simulink model "PVmpptBuckConverter"  (R2020b)
settings: Solver=FixedStepDiscrete  StartTime=0.0  StopTime=0.5  FixedStep=1e-6  RelTol=1e-3
values from neighbouring files (symbols this model uses):
  C = (Iripp)/(8*fs*Vripp)    (= 0.00025)    [BuckConverterCalculos.m]
  L = (Vout* (Vin-Vout))/ (Iripp*fs *Vin)    (= 0.0714285714286)    [BuckConverterCalculos.m]
  Ts = 1e-6    (= 1e-06)    [BuckConverterCalculos.m]
undefined symbols (not defined in the file or in its folder): Ion, Lithium
libraries: powerlib x6, powerlib_meascontrol x2, electricdrivelib x1, re_lib x1
settings Model: Creator=User  LastModifiedBy=User

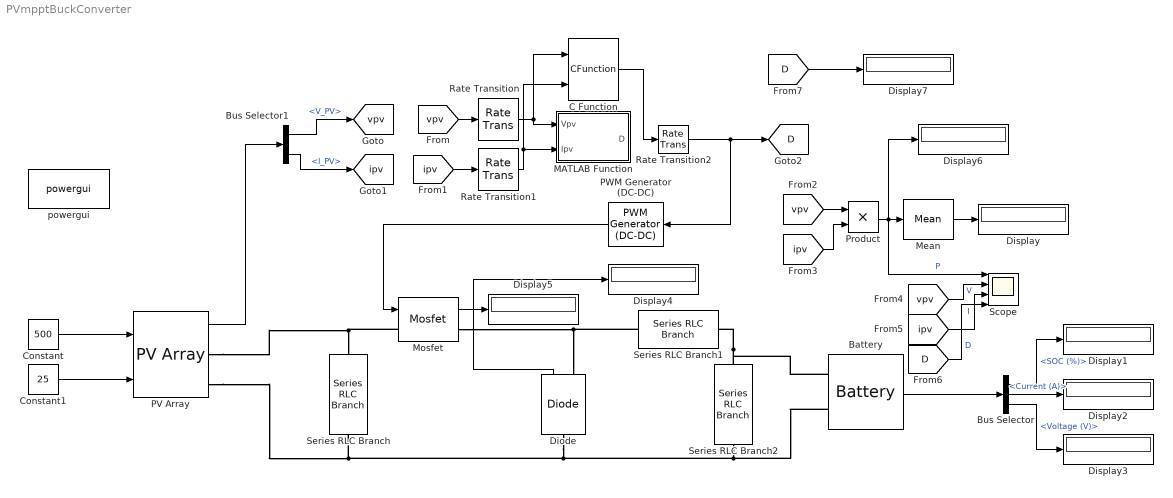
== system PVmpptBuckConverter ==
  Battery : electricdrivelib/Extra Sources/Battery  BatType=Lithium-Ion  ShowTempParam=off  ThermalPreset=no  ShowAgeParam=off  NomV=5  NomQ=50  SOC=45  Batt_Tr=1  PresetModel=on  MaxQ=50  MinV=3.75  FullV=5.8199  Dis_rate=21.7391  R=0.001  Normal_OP=45.2174  expZone="[5.4019      2.4565]"  current=[6.5 13 32.5]  Units=Time  Tci=20  NomT=20  T2=-30  MaxQ2=4.8  FullV2=7.1  Normal_OP2=5.655  expZone2="[6.58           1]"  Rca=0.6  ti=2000  Dp=0  Neq0=0  Tsim=1e6  Ta1=25  Qeol=5.4*0.9  Reol=0.013333*1.2  Char_age=[2.3478, 3]  Dis_age=[2.3478, 10]  N1=1500  N2=10500  N3=1000  N4=1400  Ta2=45  N5=950
  Bus Selector : BusSelector  OutputSignals=SOC (%),Current (A),Voltage (V)
  Bus Selector1 : BusSelector  OutputSignals=V_PV,I_PV
  C Function : CFunction  OutputCode=|  StartCode=|
      OutputCode=|
      | double Ppv = Vpv * Ipv;
      |     double delP = Ppv - Pprev;
      |     double delV = Vpv - Vprev;
      |     
      |     if (delP != 0) {
      |         if (delP > 0) {
      |             if (delV > 0) {
      |                 D = Dprev - deltaD;
      |             } else {
      |                 D = Dprev + deltaD;
      |             }
      |         } else {
      |             if (delV > 0) {
      |                 D = Dprev + deltaD;
      |             } else {
      |                 D = Dprev - deltaD;
      |             }
      |         }
      |     } else {
      |         D = Dprev;
      |     }
      |     if ((D > Dmax) || (D < Dmin)) {
      |         D = Dprev;
      |     }
      |     
      |     Dprev = D;
      |     Pprev = Ppv;
      |     Vprev = Vpv;
      StartCode=|
      | Dmin = 0.05;
      | Dmax = 0.95;
      | Dprev = 0.95;
      | Vprev = 0;
      | Pprev = 0;
      | deltaD = 0.02;
  Constant : Constant  Value=500  SampleTime=Ts
  Constant1 : Constant  Value=25  SampleTime=Ts
  Diode : powerlib/Power Electronics/Diode  Ron=0.001  Lon=0  Vf=0.8  IC=0  UseSnubber=0  Rs=500  Cs=250e-9  Measurements=on
  Display{,1..7} (8 alike) : Display
  MATLAB Function : MATLAB Function  TreatAsAtomicUnit=on
  Mean : powerlib_meascontrol/Measurements/Mean  Freq=60  Vinit=0  Ts=Ts
  Mosfet : powerlib/Power Electronics/Mosfet  Ron=0.1  Lon=0  Rd=0.01  Vfd=0  IC=0  Rs=1e5  Cs=inf  Measurements=on
  PV Array : re_lib/Solar/PV Array  Npar=1  Nser=1  PlotType=array @ 25 deg.C & specified irradiances  S_vec="[ 1000  500  100 ]"  Temp_C_vec="[ 45 25  ]"  ModuleName=User-defined  PlotWhenSelected=off  Pm=5.075  Ncell=36  Voc=22  Isc=0.32  Vm=17.5  Im=0.29  beta_Voc_pc=-0.291  alpha_Isc_pc=0.013301  beta_Voc=-0.06402  alpha_Isc=4.2563e-05  IL=0.32489  I0=6.8687e-13  nI=0.88738  Rsh=903.5702  Rs=6.9286  RobustModel=off  RobustCellTemperature=313.3991  BAL=on  Tc=1e-6  Tfilter=5e-5
  PWM Generator (DC-DC) : powerlib_meascontrol/Pulse & Signal Generators/PWM Generator (DC-DC)  Fsw=500  Ts=Ts
  Product : Product
  Rate Transition : RateTransition  OutPortSampleTime=Ts_control
  Rate Transition1 : RateTransition  OutPortSampleTime=Ts_control
  Rate Transition2 : RateTransition  OutPortSampleTime=Ts
  Scope : Scope  NumInputPorts=4
  Series RLC Branch : powerlib/Elements/Series RLC Branch  LConnTagsString=__new0  RConnTagsString=__new0  BranchType=RC  Resistance=0.001  Inductance=1e-3  SetiL0=off  InitialCurrent=0  Capacitance=C*4  Setx0=off  InitialVoltage=0  Measurements=None
  Series RLC Branch1 : powerlib/Elements/Series RLC Branch  LConnTagsString=__new0  RConnTagsString=__new0  BranchType=L  Resistance=0.001  Inductance=L  SetiL0=off  InitialCurrent=0  Capacitance=2.5e-5  Setx0=off  InitialVoltage=0  Measurements=None
  Series RLC Branch2 : powerlib/Elements/Series RLC Branch  LConnTagsString=__new0  RConnTagsString=__new0  BranchType=C  Resistance=0.001  Inductance=0.0036  SetiL0=off  InitialCurrent=0  Capacitance=C  Setx0=off  InitialVoltage=0  Measurements=None
  powergui : powerlib/powergui  Priority=1  SimulationMode=Discrete  SampleTime=Ts  frequency=60  Iterations=50  frequencyindice=0  Pbase=100e6  ErrMax=1e-4  UnitsV=kV  UnitsW=MW  buscounter=0  FunctionMessages=off  echomessages=off  EnableUseOfTLC=off  CurrentSourceSwitches=off  DisableSnubberDevices=off  DisableRonSwitches=off  DisableVfSwitches=off  DisplayEquations=off  AutomaticDiscreteSolvers=off  SolverType=Tustin/Backward Euler (TBE)  Interpol=off  ExternalGateDelay=off  methode=off  Ts=100  x0status=blocks  SPID=on  SwTol=0  HookPort=off  NonlinearTolerance=1e-4  nMaxIteration=100  ContinueOnMaxIteration=off  RestoreLinks=warning  ResistiveCurrentMeasurement=off  Frange=[0:2:500]  Ylog=off  Xlog=on  ShowGrid=off  save=off  variable=ZData  structure=0  ZoomFFT=off  StartTime=0.0  cycles=1  DisplayStyle=1  fundamental=60  FreqAxis=off  MaxFrequency=1000  frequencyindicesteady=1  RmsSteady=1  display=off
  tag scope: D=global, ipv=global, vpv=global
  wires:
  Constant/1 -> PV Array/1
  Constant1/1 -> PV Array/2
  Battery/1 -> Bus Selector/1
  PV Array/1 -> Bus Selector1/1
  Bus Selector1/1 -> [vpv]  "<V_PV>"
  Bus Selector1/2 -> [ipv]  "<I_PV>"
  [vpv] -> Rate Transition/1
  [ipv] -> Rate Transition1/1
  [vpv] -> Product/1
  [ipv] -> Product/2
  Bus Selector/1 -> Display1/1  "<SOC (%)>"
  Bus Selector/2 -> Display2/1  "<Current (A)>"
  Bus Selector/3 -> Display3/1  "<Voltage (V)>"
  Diode/1 -> Display4/1
  Mosfet/1 -> Display5/1
  Product/1 -> Display6/1, Scope/1, Mean/1  "P"
  Mean/1 -> Display/1
  [vpv] -> Scope/2  "V"
  [ipv] -> Scope/3  "I"
  PWM Generator (DC-DC)/1 -> Mosfet/1
  Rate Transition2/1 -> [D], PWM Generator (DC-DC)/1
  Rate Transition/1 -> C Function/1, MATLAB Function/1(Vpv)
  Rate Transition1/1 -> MATLAB Function/2(Ipv), C Function/2
  [D] -> Scope/4  "D"
  [D] -> Display7/1
  C Function/1 -> Rate Transition2/1
  connections:
  PV Array/RConn1 -- Mosfet/LConn1 -- Series RLC Branch/LConn1
  PV Array/RConn2 -- Battery/LConn2 -- Series RLC Branch2/RConn1 -- Diode/LConn1 -- Series RLC Branch/RConn1
  Mosfet/RConn1 -- Series RLC Branch1/LConn1 -- Diode/RConn1
  Series RLC Branch2/LConn1 -- Battery/LConn1 -- Series RLC Branch1/RConn1

== matlab function PVmpptBuckConverter/MATLAB Function ==
  data: Vpv input; D output; Ipv input
function D = mpptm(Vpv,Ipv)

Dmin = 0.05;
Dmax = 0.95;
persistent Dprev Pprev Vprev ;

if isempty(Dprev)
    Dprev = 0.95;
    Vprev = 0;
    Pprev = 0;
end
%initialize parameters
deltaD = 0.02;

% initalize measured array power
Ppv = Vpv*Ipv;

if((Ppv - Pprev) ~= 0) 
    if((Ppv - Pprev) > 0) 
        if((Vpv-Vprev) > 0) 
            D = Dprev - deltaD;
        else
            D = Dprev + deltaD;
        end
    else
        if((Vpv-Vprev) > 0)
            D = Dprev + deltaD;
        else
            D = Dprev - deltaD;
        end
    end
else
    D = Dprev;
end

%update values
if D >= Dmax || D < Dmin
    D = Dprev;
end
Dprev = D;
Vprev = Vpv;
Pprev = Ppv;
